simulink model "trial_main_sys_v1_in"  (R2015a)
settings: Solver=ode23  StartTime=0.0  StopTime=Tfin  RelTol=1e-3
undefined symbols (not defined in the file): init, K, param
settings Model: Creator=jesus  LastModifiedBy=jesus

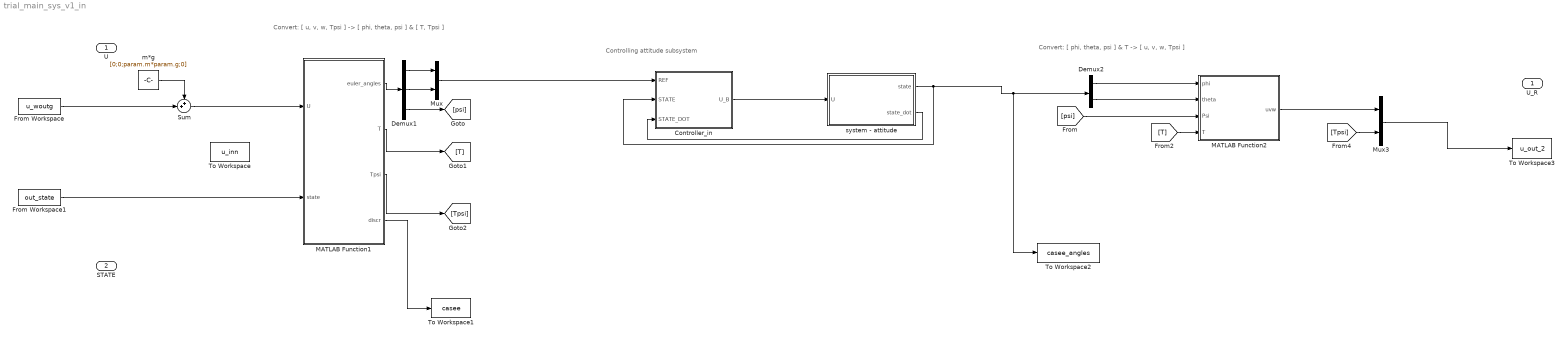
== system trial_main_sys_v1_in ==
  note: Convert:
      |  [ phi, theta, psi ] & T -> [ u, v, w, Tpsi ]
  note: Controlling attitude subsystem
  note: Convert:
      |  [ u, v, w, Tpsi ] -> [ phi, theta, psi ] & [ T, Tpsi ]
  U : Inport
  STATE : Inport  Port=2
  "Controller_in " : Subsystem
  Demux1 : Demux  Outputs=3
  Demux2 : Demux  Outputs=2
  From Workspace : FromWorkspace  VariableName=u_woutg  SampleTime=param.hf  Interpolate=off  OutputAfterFinalValue=Setting to zero
  From Workspace1 : FromWorkspace  VariableName=out_state  SampleTime=param.hf  Interpolate=off  OutputAfterFinalValue=Setting to zero
  MATLAB Function1 : MATLAB Function  TreatAsAtomicUnit=on
  MATLAB Function2 : MATLAB Function  TreatAsAtomicUnit=on
  Mux : Mux  Inputs=2
  Mux3 : Mux  Inputs=2
  Sum : Sum  Inputs=++|
  To Workspace : ToWorkspace  VariableName=u_inn  SaveFormat=Structure With Time  SampleTime=-1
  To Workspace1 : ToWorkspace  VariableName=casee  SaveFormat=Structure With Time  SampleTime=-1
  To Workspace2 : ToWorkspace  VariableName=casee_angles  SaveFormat=Structure With Time  SampleTime=-1
  To Workspace3 : ToWorkspace  VariableName=u_out_2  SaveFormat=Structure With Time  SampleTime=-1
  m*g : Constant  Value=[0;0;param.m*param.g;0]
  system - attitude : Subsystem
  U_R : Outport
  wires:
  Demux1/1 -> Mux/1
  Demux1/2 -> Mux/2
  MATLAB Function1/1(euler_angles) -> Demux1/1
  Demux1/3 -> [psi]
  MATLAB Function1/2(T) -> [T]
  "Controller_in "/1(U_B) -> system - attitude/1(U)
  [T] -> MATLAB Function2/4(T)
  [Tpsi] -> Mux3/2
  MATLAB Function2/1(uvw) -> Mux3/1
  MATLAB Function1/3(Tpsi) -> [Tpsi]
  Demux2/1 -> MATLAB Function2/1(phi)
  Demux2/2 -> MATLAB Function2/2(theta)
  [psi] -> MATLAB Function2/3(Psi)
  MATLAB Function1/4(discr) -> To Workspace1/1
  From Workspace/1 -> Sum/2
  Sum/1 -> MATLAB Function1/1(U)
  m*g/1 -> Sum/1
  From Workspace1/1 -> MATLAB Function1/2(state)
  Mux3/1 -> To Workspace3/1
  system - attitude/1(state) -> "Controller_in "/2(STATE), To Workspace2/1, Demux2/1
  Mux/1 -> "Controller_in "/1(REF)
  system - attitude/2(state_dot) -> "Controller_in "/3(STATE_DOT)

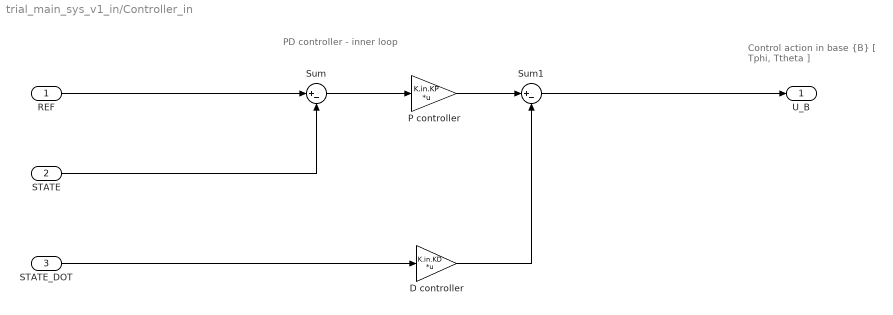
== system trial_main_sys_v1_in/Controller_in  ==
  note: Control action
      |   in base {B}
      |
      |
      |
      | [ Tphi, Ttheta ]
  note: PD controller - inner loop
  REF : Inport
  STATE : Inport  Port=2
  STATE_DOT : Inport  Port=3
  D controller : Gain  Gain=K.in.KD  Multiplication=Matrix(K*u)
  P controller : Gain  Gain=K.in.KP  Multiplication=Matrix(K*u)
  Sum : Sum  Inputs=|+-
  Sum1 : Sum  Inputs=|+-
  U_B : Outport
  wires:
  Sum1/1 -> U_B/1
  Sum/1 -> P controller/1
  P controller/1 -> Sum1/1
  REF/1 -> Sum/1
  STATE/1 -> Sum/2
  STATE_DOT/1 -> D controller/1
  D controller/1 -> Sum1/2

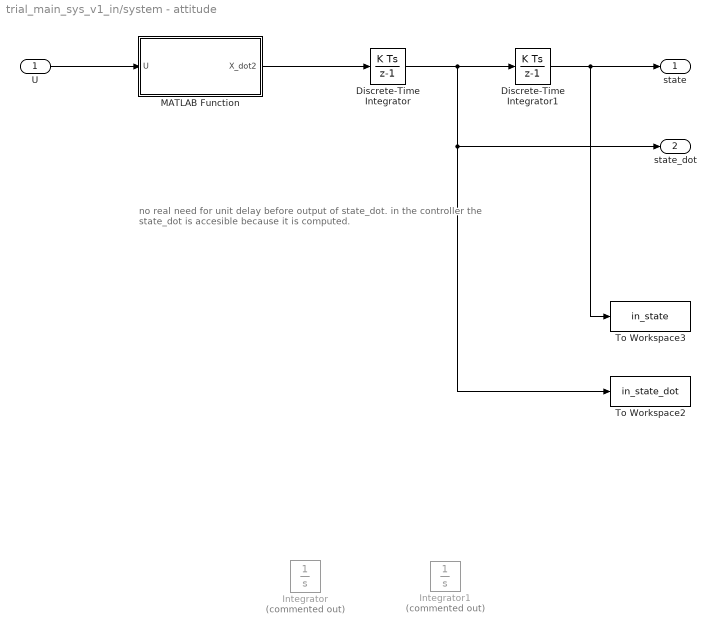
== system trial_main_sys_v1_in/system - attitude ==
  note: no real need for unit delay before output of state_dot.
      | in the controller the state_dot is accesible because it is computed.
  U : Inport
  Discrete-Time Integrator : DiscreteIntegrator  InitialConditionSetting=State (most efficient)  SampleTime=param.hf
  Discrete-Time Integrator1 : DiscreteIntegrator  InitialCondition=init.in  InitialConditionSetting=State (most efficient)  SampleTime=param.hf
  Integrator : Integrator  Commented=on  InitialCondition=[1e-7;1e-7]  ZeroCross=off
  Integrator1 : Integrator  Commented=on  InitialCondition=init.in
  MATLAB Function : MATLAB Function  TreatAsAtomicUnit=on
  To Workspace2 : ToWorkspace  VariableName=in_state_dot  SaveFormat=Structure With Time  SampleTime=-1
  To Workspace3 : ToWorkspace  VariableName=in_state  SaveFormat=Structure With Time  SampleTime=-1
  state : Outport
  state_dot : Outport  Port=2
  wires:
  U/1 -> MATLAB Function/1(U)
  MATLAB Function/1(X_dot2) -> Discrete-Time Integrator/1
  Discrete-Time Integrator1/1 -> To Workspace3/1, state/1
  Discrete-Time Integrator/1 -> state_dot/1, To Workspace2/1, Discrete-Time Integrator1/1

== matlab function trial_main_sys_v1_in/MATLAB Function1 ==
  data: U input; euler_angles output; state input; T output; Tpsi output; discr output
function [euler_angles, T, Tpsi, discr] = fcn1(U, state)

% Mathematical derivation of formulas in XXXX

% Inputs
    u_abs = U(1);   v_abs = U(2);   w_abs = U(3);
    Tpsi = U(4);
    psi = state(4);
    
% Torque
T = sqrt( u_abs^2 + v_abs^2 + w_abs^2 );

% normalization of thrust components
u = u_abs/(T);
v = v_abs/(T);
w = w_abs/(T);

% Euler angles

    % Considering w =! 0 (always true)
    %   Considering phi and theta are never 90º (iff w=!0)    

     % psi is a known value
        a = cos(psi);
        b = sin(psi);

    % compute phi & theta
    if ( u ~= 0 && v ~=0 )
        if ( a==0 )
            phi   = asin( u/b );
            theta = atan( v/(w*b) ); 
                discr = [ 1.1; u/b; v/(w*b) ];
        elseif ( b==0 )
            phi   = asin( -v/a );
            theta = atan( u/(w*a) );
                discr = [ 1.2; -v/a; u/(w*a) ];
        else
            aux = (u-v*w) / (b*(1+w));
            phi   = asin( aux );
            theta = atan ( (u-b*aux) / (w*a) );
                discr = [ 1.3; aux; (u-b*aux) / (w*a) ];
        end

    elseif ( u == 0 && v == 0 )
        phi   = 0;
        theta = 0;
            discr = [ 2; 0; 0 ];

    elseif ( u == 0 && v ~= 0 )
        if ( a==0 )
            phi   = 0;
            theta = atan ( v/(b*w) );
                discr = [ 3.1; 0; v/(b*w) ];
        elseif ( b==0 )
            phi   = asin( -v/a );
            theta = 0;
                discr = [ 3.2; -v/a; 0 ];
        else
            phi   = asin( -a*v );
            theta = atan( b*v/w );
                discr = [ 3.3; -a*v; b*v/w ];
        end

    elseif ( u ~=0 && v == 0 )
        if ( a==0 )
            phi   = asin( u/b );
            theta = 0;
                discr = [ 4.1; b/u; 0 ];
        elseif ( b==0 )
            phi   = 0;
            theta = atan( u/(a*w) );
                discr = [ 4.2; 0; u/(a*w) ];
        else 
            phi   = asin( b*u );
            theta = atan( a*u/w );
                discr = [ 4.3; u/b; a*u/w ];
        end
    else
        phi = pi/3;
        theta = pi/3;
            discr = [ 5; pi/3; pi/3 ];
    end
        euler_angles = [phi; theta; psi];
end

% 
% function [ angle ] = asinn( aa )
%     angle = asin(aa);
%     % angle correction
%     if ~( -pi/2 < angle < pi/2 )
%         angle = angle - pi/2;
%     end
% end
% 
% function [ angle ] = atann( aa )
%     angle = atan(aa);
%     % angle correction
%     if ~( -pi/2 < angle < pi/2 )
%         angle = angle - pi/2;
%     end
% end

% function [angle] = asinn( bb )
% angle = real( asin( complex(bb) ) );
% end
% 
% function [angle] = atann( bb )
% angle = real( atan( complex(bb) ) );
% end

== matlab function trial_main_sys_v1_in/MATLAB Function2 ==
  data: phi input; theta input; Psi input; uvw output; T input
function uvw  = fnc2(phi, theta, Psi, T)

% call RT2uvw

% inputs
%     phi   = euler(1);
%     theta = euler(2);
%     Psi   = euler(3);
    
% rotation matrix
    R = [cos(theta)*cos(Psi),  sin(phi)*sin(theta)*cos(Psi)-cos(phi)*sin(Psi),  cos(phi)*sin(theta)*cos(Psi)+sin(phi)*sin(Psi);
         cos(theta)*sin(Psi),  sin(phi)*sin(theta)*sin(Psi)+cos(phi)*cos(Psi),  cos(phi)*sin(theta)*sin(Psi)-sin(phi)*cos(Psi);
         -sin(theta),          sin(phi)*cos(theta),                             cos(phi)*cos(theta)                           ];

    
    
%     uvw = eul2rotm( euler_angles' ) * [0;0;T];
%uvw = [];
uvw = zeros(3,1);
uvw = R*[0; 0; T];

== matlab function trial_main_sys_v1_in/system - attitude/MATLAB Function ==
  data: U input; X_dot2 output
function X_dot2   = sys_in ( U )
%#codegen
% parameters
    Ix = 0.002237568100000;   
    Iy = 0.002985236000000;

X_dot2 = [ 0; 0];
X_dot2(1) = U(1) / Ix;
X_dot2(2) = U(2) / Iy;
